simulink model "lab 4"  (R2025a)
settings: Solver=VariableStepAuto  StartTime=0.0  StopTime=0.04  RelTol=1e-3
undefined symbols (not defined in the file): alpha
libraries: spsThyristorLib x8, spsACVoltageSourceLib x4, spsVoltageMeasurementLib x2, sps_lib x2, spsControlledCurrentSourceLib x1, spsGroundLib x1, spsMeanLib x1, spsRMSLib x1, spsSeriesRLCBranchLib x1
settings Model: Creator=088a2  LastModifiedBy=088a2

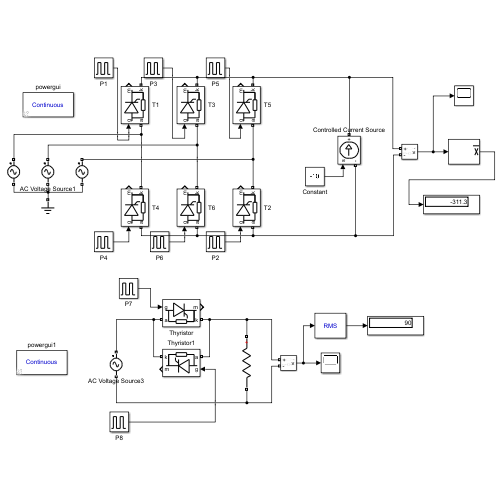
[thumbnail: Simulink's stored preview of the top-level diagram]
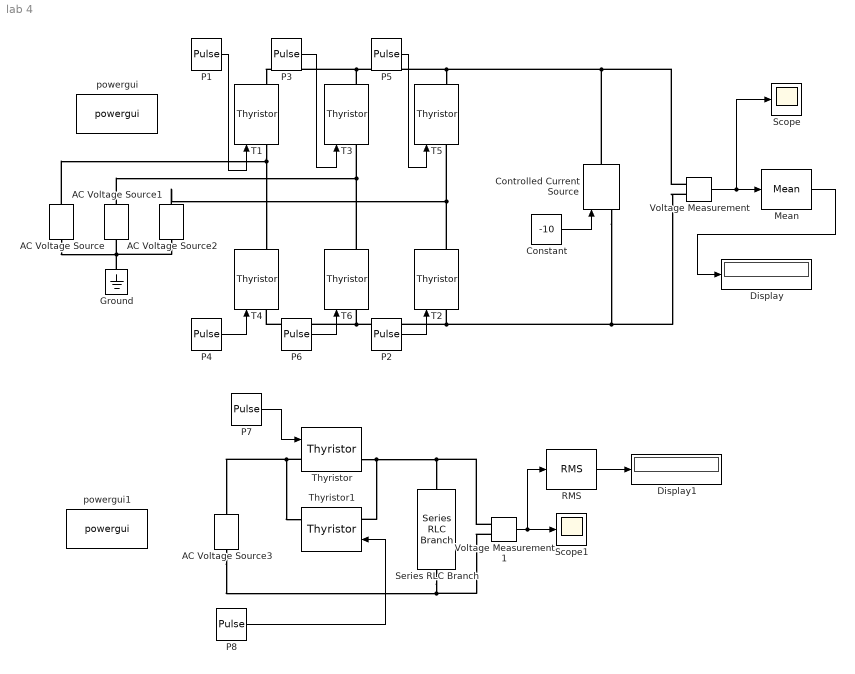
== system lab 4 ==
  AC Voltage Source : spsACVoltageSourceLib/AC Voltage Source  Amplitude=325  Phase=0  Frequency=50  SampleTime=0  Measurements=None  BusType=swing  Pref=10e3  Qref=0  Qmin=-inf  Qmax=+inf
  AC Voltage Source1 : spsACVoltageSourceLib/AC Voltage Source  Amplitude=325  Phase=-120  Frequency=50  SampleTime=0  Measurements=None  BusType=swing  Pref=10e3  Qref=0  Qmin=-inf  Qmax=+inf
  AC Voltage Source2 : spsACVoltageSourceLib/AC Voltage Source  Amplitude=325  Phase=-240  Frequency=50  SampleTime=0  Measurements=None  BusType=swing  Pref=10e3  Qref=0  Qmin=-inf  Qmax=+inf
  AC Voltage Source3 : spsACVoltageSourceLib/AC Voltage Source  Amplitude=325  Phase=0  Frequency=50  SampleTime=0  Measurements=None  BusType=swing  Pref=10e3  Qref=0  Qmin=-inf  Qmax=+inf
  Constant : Constant  Value=-10
  Controlled Current Source : spsControlledCurrentSourceLib/Controlled Current Source  Initialize=on  Source_Type=AC  Amplitude=0  Phase=0  Frequency=0  Measurements=None
  Display : Display
  Display1 : Display
  Ground : spsGroundLib/Ground  LConnTagsString=a
  Mean : spsMeanLib/Mean  Freq=50  Vinit=0  Ts=0
  P1 : DiscretePulseGenerator  PulseType=Time based  Period=0.02  PulseWidth=120/360 * 100  PhaseDelay=(alpha + 30) / 360 * 0.02
  P2 : DiscretePulseGenerator  PulseType=Time based  Period=0.02  PulseWidth=120/360 * 100  PhaseDelay=(alpha + 30 + 60) / 360 * 0.02
  P3 : DiscretePulseGenerator  PulseType=Time based  Period=0.02  PulseWidth=120/360 * 100  PhaseDelay=(alpha + 30 + 120) / 360 * 0.02
  P4 : DiscretePulseGenerator  PulseType=Time based  Period=0.02  PulseWidth=120/360 * 100  PhaseDelay=(alpha + 30 + 180) / 360 * 0.02
  P5 : DiscretePulseGenerator  PulseType=Time based  Period=0.02  PulseWidth=120/360 * 100  PhaseDelay=(alpha + 30 - 120 )/ 360 * 0.02
  P6 : DiscretePulseGenerator  PulseType=Time based  Period=0.02  PulseWidth=120/360 * 100  PhaseDelay=(alpha + 30 - 60) / 360 * 0.02
  P7 : DiscretePulseGenerator  PulseType=Time based  Period=0.02  PulseWidth=50  PhaseDelay=(alpha) / 360 * 0.02
  P8 : DiscretePulseGenerator  PulseType=Time based  Period=0.02  PulseWidth=50  PhaseDelay=(alpha + 180) / 360 * 0.02
  RMS : spsRMSLib/RMS  TrueRMS=on  Freq=50  RMSInit=0  Ts=0
  Scope : Scope
      settings: Title=230929228_Mrinal_Kumar  ActiveDisplayYMinimum=-600  ActiveDisplayYMaximum=600  YLabel=Voltage
  Scope1 : Scope
      settings: Title=230929228_Mrinal_Kumar  ActiveDisplayYMinimum=-405.20947905395383  ActiveDisplayYMaximum=405.20947905395383  YLabel=Voltage
  Series RLC Branch : spsSeriesRLCBranchLib/Series RLC Branch  LConnTagsString=__new0  RConnTagsString=__new0  BranchType=R  Resistance=10  Inductance=1e-3  SetiL0=off  InitialCurrent=0  Capacitance=1e-6  Setx0=off  InitialVoltage=0  Measurements=None
  T{1..6} (6 alike) : spsThyristorLib/Thyristor  Ron=0.001  Lon=0  Vf=0.8  IC=0  Rs=500  Cs=250e-9  Measurements=on
  Thyristor : spsThyristorLib/Thyristor  Ron=0.001  Lon=0  Vf=0.8  IC=0  Rs=500  Cs=250e-9  Measurements=on
  Thyristor1 : spsThyristorLib/Thyristor  Ron=0.001  Lon=0  Vf=0.8  IC=0  Rs=500  Cs=250e-9  Measurements=on
  Voltage Measurement : spsVoltageMeasurementLib/Voltage Measurement  PhasorSimulation=off  OutputType=Complex  PSBequivalent=0
  Voltage Measurement1 : spsVoltageMeasurementLib/Voltage Measurement  PhasorSimulation=off  OutputType=Complex  PSBequivalent=0
  powergui : sps_lib/powergui  Priority=1  SimulationMode=Continuous  SampleTime=50e-6  frequency=60  Iterations=50  frequencyindice=50  Pbase=100e6  ErrMax=1e-4  UnitsV=kV  UnitsW=MW  buscounter=0  FunctionMessages=off  echomessages=off  EnableUseOfTLC=off  CurrentSourceSwitches=off  DisableSnubberDevices=off  DisableRonSwitches=off  DisableVfSwitches=off  DisplayEquations=off  AutomaticDiscreteSolvers=off  SolverType=Tustin/Backward Euler (TBE)  Interpol=off  ExternalGateDelay=off  methode=off  Ts=100  x0status=zero  SPID=on  SwTol=0  HookPort=off  NonlinearTolerance=1e-4  nMaxIteration=100  ContinueOnMaxIteration=off  RestoreLinks=warning  ResistiveCurrentMeasurement=off  Frange=[0:2:500]  Ylog=off  Xlog=on  ShowGrid=off  save=off  variable=ZData  structure=0  ZoomFFT=off  StartTime=0.0  cycles=1  DisplayStyle=1  fundamental=60  FreqAxis=off  MaxFrequency=1000  frequencyindicesteady=1  RmsSteady=1  display=off
  powergui1 : sps_lib/powergui  Priority=1  SimulationMode=Continuous  SampleTime=50e-6  frequency=60  Iterations=50  frequencyindice=50  Pbase=100e6  ErrMax=1e-4  UnitsV=kV  UnitsW=MW  buscounter=0  FunctionMessages=off  echomessages=off  EnableUseOfTLC=off  CurrentSourceSwitches=off  DisableSnubberDevices=off  DisableRonSwitches=off  DisableVfSwitches=off  DisplayEquations=off  AutomaticDiscreteSolvers=off  SolverType=Tustin/Backward Euler (TBE)  Interpol=off  ExternalGateDelay=off  methode=off  Ts=100  x0status=zero  SPID=on  SwTol=0  HookPort=off  NonlinearTolerance=1e-4  nMaxIteration=100  ContinueOnMaxIteration=off  RestoreLinks=warning  ResistiveCurrentMeasurement=off  Frange=[0:2:500]  Ylog=off  Xlog=on  ShowGrid=off  save=off  variable=ZData  structure=0  ZoomFFT=off  StartTime=0.0  cycles=1  DisplayStyle=1  fundamental=60  FreqAxis=off  MaxFrequency=1000  frequencyindicesteady=1  RmsSteady=1  display=off
  wires:
  Constant/1 -> Controlled Current Source/1
  P1/1 -> T1/1
  P3/1 -> T3/1
  P5/1 -> T5/1
  P6/1 -> T6/1
  P2/1 -> T2/1
  Voltage Measurement/1 -> Scope/1, Mean/1
  Mean/1 -> Display/1
  P4/1 -> T4/1
  Voltage Measurement1/1 -> RMS/1, Scope1/1
  P7/1 -> Thyristor/1
  P8/1 -> Thyristor1/1
  RMS/1 -> Display1/1
  connections:
  Ground/LConn1 -- AC Voltage Source1/LConn1 -- AC Voltage Source2/LConn1 -- AC Voltage Source/LConn1
  T1/LConn1 -- AC Voltage Source/RConn1 -- T4/RConn1
  T6/RConn1 -- T3/LConn1 -- AC Voltage Source1/RConn1
  T2/RConn1 -- T5/LConn1 -- AC Voltage Source2/RConn1
  Controlled Current Source/LConn1 -- Voltage Measurement/LConn2 -- T2/LConn1 -- T6/LConn1 -- T4/LConn1
  Controlled Current Source/RConn1 -- Voltage Measurement/LConn1 -- T5/RConn1 -- T3/RConn1 -- T1/RConn1
  Thyristor/LConn1 -- Thyristor1/RConn1 -- AC Voltage Source3/RConn1
  Thyristor/RConn1 -- Voltage Measurement1/LConn1 -- Series RLC Branch/LConn1 -- Thyristor1/LConn1
  Series RLC Branch/RConn1 -- Voltage Measurement1/LConn2 -- AC Voltage Source3/LConn1
